simulink model "HVDCMTGW"  (R2025b)
settings: Solver=VariableStepAuto  StartTime=0.0  StopTime=Tsim  FixedStep=5e-5  RelTol=1e-3
PreLoadFcn:
  | SimulationTime = 3.5;
  | HVDCParameters;
  | Tsim = 3.5;
undefined symbols (not defined in the file): base, Base, Connection1, Connection2, Connection3, DiscIntNeverNeededParam, ee_sli_rtmsupport, frt, gcbh, grid, HVDC, lvrt, onshoreGfm, pll, pmsm, PVController, time, Ts, windController, windTransformer, windTurbine
libraries: fl_lib x51, ee_lib x46, nesl_utility x41, simulink x18, eeGeneralControl x12, eeTransforms x6
(part 2 of 4)

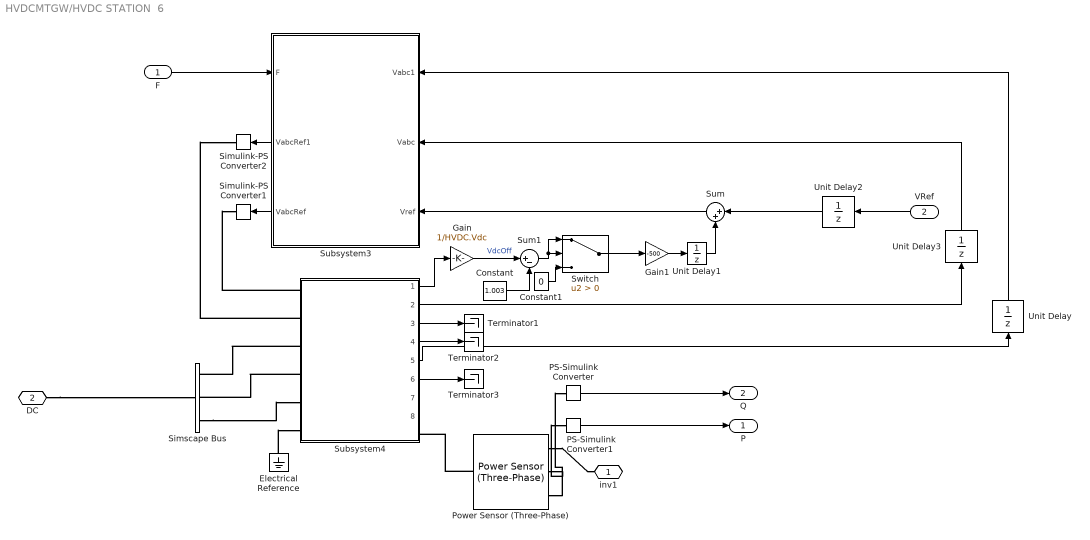
== system HVDCMTGW/HVDC STATION  6 ==
  F : Inport
  VRef : Inport  Port=2
  Constant : Constant  Value=1.003
  Constant1 : Constant  Value=0
  Electrical Reference : fl_lib/Electrical/Electrical Elements/Electrical Reference
  Gain : Gain  Gain=1/HVDC.Vdc
  Gain1 : Gain  Gain=-500
  PS-Simulink Converter : nesl_utility/PS-Simulink Converter  PhysicalDomain=network_engine_domain  SubClassName=ps_output  LeftPortType=input  RightPortType=output  PseudoPeriodic=off  Frequencies=[]  VectorFormat=inherit  Unit=inherit  AffineConversion=off
  PS-Simulink Converter1 : nesl_utility/PS-Simulink Converter  PhysicalDomain=network_engine_domain  SubClassName=ps_output  LeftPortType=input  RightPortType=output  PseudoPeriodic=off  Frequencies=[]  VectorFormat=inherit  Unit=inherit  AffineConversion=off
  Power Sensor (Three-Phase) : ee_lib/Sensors & Transducers/Power Sensor (Three-Phase)  load_type=ee.enum.passive.type_balanced.balanced  f0=60 Hz
      settings: InternalSimscapePortConfiguration="{\"Bottom\":[],\"Left\":[{\"id\":\"N1\",\"label\":\"~1\",\"type\":\"foundation.electrical.three_phase\"}],\"Right\":[{\"id\":\"N2\",\"label\":\"~2\",\"type\":\"foundation.electrical.three_phase\"}],\"Top\":[{\"id\":\"Pm\",\"label\":\"P\",\"type\":\"output\"},{\"id\":\"Qm\",\"label\":\"Q\",\"type\":\"output\"}]}"
  Simscape Bus : SimscapeBus  HierarchyStrings=Connection1;Connection2;Connection3
  Simulink-PS Converter1 : nesl_utility/Simulink-PS Converter  PhysicalDomain=network_engine_domain  SubClassName=ps_input  LeftPortType=input  RightPortType=output  PseudoPeriodic=off  Frequencies=[]  NoiseDistribution=none  NoiseParameters=[]  Unit=1  AffineConversion=off  FilteringAndDerivatives=provide  SimscapeFilterOrder=1  InputFilterTimeConstant=0.001  UdotUserProvided=0
  Simulink-PS Converter2 : nesl_utility/Simulink-PS Converter  PhysicalDomain=network_engine_domain  SubClassName=ps_input  LeftPortType=input  RightPortType=output  PseudoPeriodic=off  Frequencies=[]  NoiseDistribution=none  NoiseParameters=[]  Unit=1  AffineConversion=off  FilteringAndDerivatives=provide  SimscapeFilterOrder=1  InputFilterTimeConstant=0.001  UdotUserProvided=0
  Subsystem3 : Subsystem
      settings: PortSchema="{\"entries\":[{\"content\":{\"sides\":[{\"content\":{\"connectorIds\":[\"In1\",\"In2\",\"In3\"]},\"type\":\"ConnectorPlacement.EquallySpacedRectSide\",\"uuid\":\"fdf47ade-06a3-4164-a0ae-b5ab8f0b8a55\"},{\"content\":{\"connectorIds\":[\"In4\",\"Out1\",\"Out2\"],\"side\":\"RIGHT\"},\"type\":\"ConnectorPlacement.EquallySpacedRectSide\",\"uuid\":\"e0a966ff-b656-4cbf-a7ff-a400da725053\"},{\"content\":{\"side\":\"TOP\"},\"type\":\"ConnectorPlacement.EquallySpacedRectSide\",\"uuid\":\"151062ed-8c36-492f-8148-99554d7644ec\"},{\"content\":{\"side\":\"BOTTOM\"},\"type\":\"ConnectorPlacement.EquallySpacedRectSide\",\"uuid\":\"8f8a2450-c04a-404e-aef9-a0f993b87536\"}]},\"type\":\"ConnectorPlacement.EquallySpacedConnector\",\"uuid\":\"01811104-26cd-432b-92b8-9bb1e91d8204\"}],\"packageUris\":[\"http://schema.mathworks.com/mf0/Connector/R2020b\"],\"version\":\"1.0\"}"
  Subsystem4 : Subsystem  ReferencedSubsystem=HVDCSTATION  c=HVDC.C*0.1  vc=HVDC.Vdc  L=HVDC.L/5  VRated=base.kV1  SRated=Base.MVA_base_new  t=grid.sensorTime  Ts=Ts
  Sum : Sum  Inputs=|++
  Sum1 : Sum  Inputs=|+-
  Switch : Switch  Criteria=u2 > Threshold  SaturateOnIntegerOverflow=off  InputSameDT=off
  Terminator1 : Terminator
  Terminator2 : Terminator
  Terminator3 : Terminator
  Unit Delay{,1..3} (4 alike) : UnitDelay  SampleTime=-1  HasFrameUpgradeWarning=on
  inv1 : PMIOPort  Side=Right
  DC : PMIOPort  Port=2  Side=Left
  P : Outport
  Q : Outport  Port=2
  wires:
  VRef/1 -> Unit Delay2/1
  Subsystem4/4 -> Terminator2/1
  F/1 -> Subsystem3/4(F)
  Subsystem4/2 -> Unit Delay3/1
  Unit Delay/1 -> Subsystem3/1(Vabc1)
  Subsystem4/3 -> Terminator1/1
  Subsystem4/5 -> Unit Delay/1
  Unit Delay3/1 -> Subsystem3/2(Vabc)
  Subsystem4/6 -> Terminator3/1
  Sum/1 -> Subsystem3/3(Vref)
  Subsystem4/1 -> Gain/1
  Unit Delay1/1 -> Sum/2
  Gain1/1 -> Unit Delay1/1
  Gain/1 -> Sum1/1  "VdcOff"
  Constant/1 -> Sum1/2
  Sum1/1 -> Switch/1, Switch/2
  Constant1/1 -> Switch/3
  Switch/1 -> Gain1/1
  PS-Simulink Converter/1 -> Q/1
  PS-Simulink Converter1/1 -> P/1
  Unit Delay2/1 -> Sum/1
  Subsystem3/1(VabcRef1) -> Simulink-PS Converter2/1
  Subsystem3/2(VabcRef) -> Simulink-PS Converter1/1
  connections:
  DC/RConn1 -- Simscape Bus/RConn1
  Subsystem4/LConn3 -- Simscape Bus/LConn1
  Power Sensor (Three-Phase)/LConn1 -- inv1/RConn1
  Power Sensor (Three-Phase)/RConn1 -- Subsystem4/RConn1
  Subsystem4/LConn4 -- Simscape Bus/LConn2
  Simscape Bus/LConn3 -- Subsystem4/LConn5
  Power Sensor (Three-Phase)/LConn3 -- PS-Simulink Converter/LConn1
  Power Sensor (Three-Phase)/LConn2 -- PS-Simulink Converter1/LConn1
  Electrical Reference/LConn1 -- Subsystem4/LConn6
  Subsystem4/LConn1 -- Simulink-PS Converter1/RConn1
  Subsystem4/LConn2 -- Simulink-PS Converter2/RConn1

== system HVDCMTGW/HVDC STATION 1 ==
  QRef1 : Inport
  QRef : Inport  Port=2
  vdcRef : Inport  Port=3
  vdcRef1 : Inport  Port=4
  PS Terminator : fl_lib/Physical Signals/Sinks/PS Terminator
  Simscape Bus : SimscapeBus  HierarchyStrings=Connection1;Connection2;Connection3
  Simulink-PS Converter1 : nesl_utility/Simulink-PS Converter  PhysicalDomain=network_engine_domain  SubClassName=ps_input  LeftPortType=input  RightPortType=output  PseudoPeriodic=off  Frequencies=[]  NoiseDistribution=none  NoiseParameters=[]  Unit=1  AffineConversion=off  FilteringAndDerivatives=provide  SimscapeFilterOrder=1  InputFilterTimeConstant=0.001  UdotUserProvided=0
  Simulink-PS Converter2 : nesl_utility/Simulink-PS Converter  PhysicalDomain=network_engine_domain  SubClassName=ps_input  LeftPortType=input  RightPortType=output  PseudoPeriodic=off  Frequencies=[]  NoiseDistribution=none  NoiseParameters=[]  Unit=1  AffineConversion=off  FilteringAndDerivatives=provide  SimscapeFilterOrder=1  InputFilterTimeConstant=0.001  UdotUserProvided=0
  Subsystem : Subsystem  ReferencedSubsystem=DCVoltageControl  Kppll=PLL.Kp_pll  Kipll=PLL.Ki_pll  frequency=Grid.frequency  initialPhase=0  sampleTime=-1  Kpicd=PVController.Kp_ic*1.02  Kiicd=PVController.Ki_ic*2  Kdicd=.5  Kpicq=PVController.Kp_ic  Kiicq=PVController.Ki_ic*2  Kdicq=.5  Kpv=20  Kiv=1000  Kdv=0  L=HVDC.L*5  iMax=HVDC.Imaxpu  zBase=Base.z_base  mVAbase=Base.MVA_base_new  VdcBase=HVDC.Vdcbase
  Subsystem1 : Subsystem  ReferencedSubsystem=DCVoltageControl  Kppll=PLL.Kp_pll  Kipll=PLL.Ki_pll  frequency=Grid.frequency  initialPhase=0  sampleTime=-1  Kpicd=PVController.Kp_ic*1.02  Kiicd=PVController.Ki_ic*2  Kdicd=0.5  Kpicq=PVController.Kp_ic  Kiicq=PVController.Ki_ic*2  Kdicq=0.5  Kpv=20  Kiv=1000  Kdv=0  L=HVDC.L*5  iMax=HVDC.Imaxpu  zBase=Base.z_base  mVAbase=Base.MVA_base_new  VdcBase=HVDC.Vdcbase
  Subsystem2 : Subsystem  ReferencedSubsystem=HVDCSTATION  c=HVDC.C*0.175  vc=HVDC.Vdc  L=HVDC.L*100  VRated=Base.KV_base_new  SRated=Base.MVA_base_new  t=Grid.sensor_time  Ts=Ts
  Subsystem3 : Subsystem
  Unit Delay1 : UnitDelay  SampleTime=Ts  HasFrameUpgradeWarning=on
  Unit Delay2 : UnitDelay  SampleTime=Ts  HasFrameUpgradeWarning=on
  DC : PMIOPort  Side=Left
  inv1 : PMIOPort  Port=2  Side=Right
  Idc : PMIOPort  Port=3  Side=Left
  wires:
  Unit Delay1/1 -> Simulink-PS Converter1/1
  Unit Delay2/1 -> Simulink-PS Converter2/1
  Subsystem/1 -> Unit Delay2/1
  Subsystem1/1 -> Unit Delay1/1
  vdcRef/1 -> Subsystem/4
  QRef/1 -> Subsystem/5
  vdcRef1/1 -> Subsystem1/4
  QRef1/1 -> Subsystem1/5
  Subsystem2/1 -> Subsystem/1
  Subsystem2/2 -> Subsystem/2
  Subsystem2/3 -> Subsystem/3
  Subsystem2/4 -> Subsystem1/1
  Subsystem2/5 -> Subsystem1/2
  Subsystem2/6 -> Subsystem1/3
  connections:
  Subsystem2/RConn1 -- inv1/RConn1
  Subsystem2/LConn2 -- Simulink-PS Converter1/RConn1
  Subsystem2/LConn1 -- Simulink-PS Converter2/RConn1
  DC/RConn1 -- Simscape Bus/RConn1
  Simscape Bus/LConn2 -- Subsystem3/RConn4 -- Subsystem2/LConn4
  Subsystem3/RConn3 -- Simscape Bus/LConn1
  Subsystem3/LConn1 -- Subsystem2/LConn3
  Idc/RConn1 -- Subsystem3/RConn1
  PS Terminator/LConn1 -- Subsystem3/RConn2
  Simscape Bus/LConn3 -- Subsystem2/LConn5

== system HVDCMTGW/HVDC STATION 2 ==
  QRef1 : Inport
  QRef : Inport  Port=2
  vdcRef1 : Inport  Port=3
  vdcRef : Inport  Port=4
  Bus Selector : BusSelector  OutputSignals=Vmag [pu],f
  Gain : Gain
  PS Terminator : fl_lib/Physical Signals/Sinks/PS Terminator
  Simscape Bus : SimscapeBus  HierarchyStrings=Connection1;Connection2;Connection3
  Simulink-PS Converter1 : nesl_utility/Simulink-PS Converter  PhysicalDomain=network_engine_domain  SubClassName=ps_input  LeftPortType=input  RightPortType=output  PseudoPeriodic=off  Frequencies=[]  NoiseDistribution=none  NoiseParameters=[]  Unit=1  AffineConversion=off  FilteringAndDerivatives=provide  SimscapeFilterOrder=1  InputFilterTimeConstant=0.001  UdotUserProvided=0
  Simulink-PS Converter2 : nesl_utility/Simulink-PS Converter  PhysicalDomain=network_engine_domain  SubClassName=ps_input  LeftPortType=input  RightPortType=output  PseudoPeriodic=off  Frequencies=[]  NoiseDistribution=none  NoiseParameters=[]  Unit=1  AffineConversion=off  FilteringAndDerivatives=provide  SimscapeFilterOrder=1  InputFilterTimeConstant=0.001  UdotUserProvided=0
  Subsystem : Subsystem  ReferencedSubsystem=DCVoltageControl  Kppll=PLL.Kp_pll  Kipll=PLL.Ki_pll  frequency=Grid.frequency  initialPhase=0  sampleTime=-1  Kpicd=PVController.Kp_ic*1.02  Kiicd=PVController.Ki_ic*2  Kdicd=.5  Kpicq=PVController.Kp_ic  Kiicq=PVController.Ki_ic*2  Kdicq=.5  Kpv=20  Kiv=1000  Kdv=0  L=HVDC.L*5  iMax=HVDC.Imaxpu  zBase=Base.z_base  mVAbase=Base.MVA_base_new  VdcBase=HVDC.Vdcbase
  Subsystem1 : Subsystem  ReferencedSubsystem=DCVoltageControl  Kppll=PLL.Kp_pll  Kipll=PLL.Ki_pll  frequency=Grid.frequency  initialPhase=0  sampleTime=-1  Kpicd=PVController.Kp_ic*1.02  Kiicd=PVController.Ki_ic*2  Kdicd=0.5  Kpicq=PVController.Kp_ic  Kiicq=PVController.Ki_ic*2  Kdicq=0.5  Kpv=20  Kiv=1000  Kdv=0  L=HVDC.L*5  iMax=HVDC.Imaxpu  zBase=Base.z_base  mVAbase=Base.MVA_base_new  VdcBase=HVDC.Vdcbase
  Subsystem2 : Subsystem  ReferencedSubsystem=HVDCSTATION  c=HVDC.C*0.175  vc=HVDC.Vdc  L=HVDC.L*100  VRated=Base.KV_base_new  SRated=Base.MVA_base_new  t=Grid.sensor_time  Ts=Ts
  Subsystem3 : Subsystem
  Terminator : Terminator
  Terminator1 : Terminator
  To Workspace1 : ToWorkspace  VariableName=f  SaveFormat=Timeseries  SampleTime=-1
  To Workspace3 : ToWorkspace  VariableName=Vmag  SaveFormat=Timeseries  SampleTime=-1
  Unit Delay1 : UnitDelay  SampleTime=Ts  HasFrameUpgradeWarning=on
  Unit Delay2 : UnitDelay  SampleTime=Ts  HasFrameUpgradeWarning=on
  Idc : PMIOPort  Side=Left
  DC : PMIOPort  Port=2  Side=Left
  inv1 : PMIOPort  Port=3  Side=Right
  wires:
  Unit Delay1/1 -> Simulink-PS Converter1/1
  Unit Delay2/1 -> Simulink-PS Converter2/1
  Subsystem/1 -> Unit Delay2/1
  Subsystem1/1 -> Unit Delay1/1
  vdcRef/1 -> Subsystem/4
  QRef/1 -> Subsystem/5
  vdcRef1/1 -> Subsystem1/4
  QRef1/1 -> Subsystem1/5
  Subsystem2/1 -> Subsystem/1
  Subsystem2/2 -> Subsystem/2
  Subsystem2/3 -> Subsystem/3
  Subsystem2/4 -> Subsystem1/1
  Subsystem2/5 -> Subsystem1/2
  Subsystem2/6 -> Subsystem1/3
  Subsystem/2 -> Bus Selector/1
  Bus Selector/1 -> To Workspace3/1, Terminator/1  "<Vmag [pu]>"
  Bus Selector/2 -> Gain/1, Terminator1/1  "<f>"
  Gain/1 -> To Workspace1/1
  connections:
  Subsystem2/RConn1 -- inv1/RConn1
  Subsystem2/LConn2 -- Simulink-PS Converter1/RConn1
  Subsystem2/LConn1 -- Simulink-PS Converter2/RConn1
  Simscape Bus/LConn3 -- Subsystem2/LConn5
  DC/RConn1 -- Simscape Bus/RConn1
  Simscape Bus/LConn2 -- Subsystem3/RConn4 -- Subsystem2/LConn4
  Subsystem3/RConn3 -- Simscape Bus/LConn1
  Idc/RConn1 -- Subsystem3/RConn1
  Subsystem3/LConn1 -- Subsystem2/LConn3
  PS Terminator/LConn1 -- Subsystem3/RConn2

== system HVDCMTGW/HVDC STATION 3 ==
  QRef : Inport
  QRef1 : Inport  Port=2
  vdcRef : Inport  Port=3
  vdcRef1 : Inport  Port=4
  GFL Control : Subsystem  VariantControl=Choice==1
      mask Display:
      | text(40,10, 'Grid Following');
      | image('HVDCstation1.png', [0,2,12,2,80,80]);
  GFM Control : Subsystem  VariantControl=Choice==2
      mask Display:
      | text(40,10, 'Grid Forming');
      | image('HVDCstation1.png', [0,2,12,2,80,80]);
  Idc : PMIOPort  Side=Left
  DC : PMIOPort  Port=2  Side=Left
  inv1 : PMIOPort  Port=3  Side=Right

== system HVDCMTGW/Subsystem ==
  Pm : Inport
  Pref : Inport  Port=2
  Constant : Constant  Value=f
  Gain : Gain  Gain=kp
  Lead-Lag (Discrete or Continuous) : eeGeneralControl/Lead-Lag (Discrete or Continuous)  T1=0  T2=t  B=inf  A=-inf  init_option=Inherited from block input  x0=0  Ts=-1
      settings: LibrarySourceBlock=|
      | ee_sl_lib/General Control/Lead-Lag
      | (Discrete or Continuous)
  Sum : Sum  Inputs=|+-
  Sum1 : Sum  Inputs=|++
  f : Outport
  wires:
  Pref/1 -> Sum/1
  Sum/1 -> Gain/1
  Pm/1 -> Lead-Lag (Discrete or Continuous)/1
  Constant/1 -> Sum1/2
  Sum1/1 -> f/1
  Lead-Lag (Discrete or Continuous)/1 -> Sum/2
  Gain/1 -> Sum1/1

== system HVDCMTGW/Subsystem1 ==
  Qm : Inport
  Qref : Inport  Port=2
  Constant : Constant  Value=V
  Gain : Gain  Gain=kq
  Lead-Lag (Discrete or Continuous) : eeGeneralControl/Lead-Lag (Discrete or Continuous)  T1=0  T2=t  B=inf  A=-inf  init_option=Inherited from block input  x0=0  Ts=-1
      settings: LibrarySourceBlock=|
      | ee_sl_lib/General Control/Lead-Lag
      | (Discrete or Continuous)
  Sum : Sum  Inputs=|+-
  Sum1 : Sum  Inputs=|++
  V : Outport
  wires:
  Qref/1 -> Sum/1
  Sum/1 -> Gain/1
  Qm/1 -> Lead-Lag (Discrete or Continuous)/1
  Constant/1 -> Sum1/2
  Sum1/1 -> V/1
  Lead-Lag (Discrete or Continuous)/1 -> Sum/2
  Gain/1 -> Sum1/1

== system HVDCMTGW/Subsystem2 ==
  Pm : Inport
  Pref : Inport  Port=2
  Constant : Constant  Value=f
  Gain : Gain  Gain=kp
  Lead-Lag (Discrete or Continuous) : eeGeneralControl/Lead-Lag (Discrete or Continuous)  T1=0  T2=t  B=inf  A=-inf  init_option=Inherited from block input  x0=0  Ts=-1
      settings: LibrarySourceBlock=|
      | ee_sl_lib/General Control/Lead-Lag
      | (Discrete or Continuous)
  Sum : Sum  Inputs=|+-
  Sum1 : Sum  Inputs=|++
  f : Outport
  wires:
  Pref/1 -> Sum/1
  Sum/1 -> Gain/1
  Pm/1 -> Lead-Lag (Discrete or Continuous)/1
  Constant/1 -> Sum1/2
  Sum1/1 -> f/1
  Gain/1 -> Sum1/1
  Lead-Lag (Discrete or Continuous)/1 -> Sum/2

== system HVDCMTGW/Subsystem3 ==
  Qm : Inport
  Qref : Inport  Port=2
  Constant : Constant  Value=V
  Gain : Gain  Gain=kq
  Lead-Lag (Discrete or Continuous) : eeGeneralControl/Lead-Lag (Discrete or Continuous)  T1=0  T2=t  B=inf  A=-inf  init_option=Inherited from block input  x0=0  Ts=-1
      settings: LibrarySourceBlock=|
      | ee_sl_lib/General Control/Lead-Lag
      | (Discrete or Continuous)
  Sum : Sum  Inputs=|+-
  Sum1 : Sum  Inputs=|++
  V : Outport
  wires:
  Qref/1 -> Sum/1
  Sum/1 -> Gain/1
  Constant/1 -> Sum1/2
  Qm/1 -> Lead-Lag (Discrete or Continuous)/1
  Gain/1 -> Sum1/1
  Sum1/1 -> V/1
  Lead-Lag (Discrete or Continuous)/1 -> Sum/2

== system HVDCMTGW/Wind Farm 1 ==
  AC Cable (Three-Phase) : ee_lib/Passive/Lines/AC Cable (Three-Phase)  l=2 km  gmr=5 mm  srad=10 mm  cablerad=20 mm  Dab=25 mm  formation=1  Ra=1 Ohm/km  Rs=10 Ohm/km  epsr=2.4  epsr_env=1  prm=1  f=60 Hz  rho=100 Ohm*m  De=1 km  Rg=0.1 Ohm/km
      settings: InternalSimscapePortConfiguration="{\"Bottom\":[],\"Left\":[{\"id\":\"S1\",\"label\":\"~S1\",\"type\":\"foundation.electrical.three_phase\"},{\"id\":\"N1\",\"label\":\"~N1\",\"type\":\"foundation.electrical.three_phase\"},{\"id\":\"g1\",\"label\":\"g1\",\"type\":\"foundation.electrical.electrical\"}],\"Right\":[{\"id\":\"S2\",\"label\":\"~S2\",\"type\":\"foundation.electrical.three_phase\"},{\"id\":\"N2\",\"label\":\"~N2\",\"type\":\"foundation.electrical.three_phase\"},{\"id\":\"g2\",\"label\":\"g2\",\"type\":\"foundation.electrical.electrical\"}],\"Top\":[]}"
  Electrical Reference : fl_lib/Electrical/Electrical Elements/Electrical Reference
  Electrical Reference1 : fl_lib/Electrical/Electrical Elements/Electrical Reference
  PLL & Measurements : Subsystem
      settings: PortSchema="{\"entries\":[{\"content\":{\"sides\":[{\"content\":{\"connectorIds\":[\"Out1\",\"In1\",\"In2\"]},\"type\":\"ConnectorPlacement.EquallySpacedRectSide\",\"uuid\":\"76485780-20fe-4fcf-8224-69648da6ed2a\"},{\"content\":{\"side\":\"RIGHT\"},\"type\":\"ConnectorPlacement.EquallySpacedRectSide\",\"uuid\":\"f19a6390-e634-42c7-8d46-4cd80cbab182\"},{\"content\":{\"side\":\"TOP\"},\"type\":\"ConnectorPlacement.EquallySpacedRectSide\",\"uuid\":\"87682f72-1844-428e-be70-ad7ca3191ee3\"}]},\"type\":\"ConnectorPlacement.EquallySpacedConnector\",\"uuid\":\"f2136b07-48ec-402b-adb3-18c0bac2157c\"}],\"packageUris\":[\"http://schema.mathworks.com/mf0/Connector/R2020b\"],\"version\":\"1.0\"}"
      mask Display: image('measurements.png'); % Use "Edit Image" on toolstrip to change.
  Wind Farm : Subsystem  Variant=on  mask{Choice1=Abstract}
      mask prompts: Choice1 "Wind Farm Model"
  abc : PMIOPort  Side=Right
  wires:
  PLL & Measurements/1(Vbus) -> Wind Farm/1(Vbus)
  Wind Farm/1(Vabc) -> PLL & Measurements/1(V)
  Wind Farm/2(Iabc) -> PLL & Measurements/2(Ig)
  connections:
  Electrical Reference/LConn1 -- AC Cable (Three-Phase)/LConn3
  Electrical Reference1/LConn1 -- AC Cable (Three-Phase)/RConn3
  AC Cable (Three-Phase)/LConn2 -- abc/RConn1
  Wind Farm/RConn1 -- Wind Farm/RConn2 -- AC Cable (Three-Phase)/RConn2

== system HVDCMTGW/Wind Farm 2 ==
  AC Cable (Three-Phase) : ee_lib/Passive/Lines/AC Cable (Three-Phase)  l=2 km  gmr=5 mm  srad=10 mm  cablerad=20 mm  Dab=25 mm  formation=1  Ra=1 Ohm/km  Rs=10 Ohm/km  epsr=2.4  epsr_env=1  prm=1  f=60 Hz  rho=100 Ohm*m  De=1 km  Rg=0.1 Ohm/km
      settings: InternalSimscapePortConfiguration="{\"Bottom\":[],\"Left\":[{\"id\":\"S1\",\"label\":\"~S1\",\"type\":\"foundation.electrical.three_phase\"},{\"id\":\"N1\",\"label\":\"~N1\",\"type\":\"foundation.electrical.three_phase\"},{\"id\":\"g1\",\"label\":\"g1\",\"type\":\"foundation.electrical.electrical\"}],\"Right\":[{\"id\":\"S2\",\"label\":\"~S2\",\"type\":\"foundation.electrical.three_phase\"},{\"id\":\"N2\",\"label\":\"~N2\",\"type\":\"foundation.electrical.three_phase\"},{\"id\":\"g2\",\"label\":\"g2\",\"type\":\"foundation.electrical.electrical\"}],\"Top\":[]}"
  AC Cable (Three-Phase)1 : ee_lib/Passive/Lines/AC Cable (Three-Phase)  l=5 km  gmr=5 mm  srad=10 mm  cablerad=20 mm  Dab=25 mm  formation=1  Ra=1 Ohm/km  Rs=10 Ohm/km  epsr=2.4  epsr_env=1  prm=1  f=60 Hz  rho=100 Ohm*m  De=1 km  Rg=0.1 Ohm/km
      settings: InternalSimscapePortConfiguration="{\"Bottom\":[],\"Left\":[{\"id\":\"S1\",\"label\":\"~S1\",\"type\":\"foundation.electrical.three_phase\"},{\"id\":\"N1\",\"label\":\"~N1\",\"type\":\"foundation.electrical.three_phase\"},{\"id\":\"g1\",\"label\":\"g1\",\"type\":\"foundation.electrical.electrical\"}],\"Right\":[{\"id\":\"S2\",\"label\":\"~S2\",\"type\":\"foundation.electrical.three_phase\"},{\"id\":\"N2\",\"label\":\"~N2\",\"type\":\"foundation.electrical.three_phase\"},{\"id\":\"g2\",\"label\":\"g2\",\"type\":\"foundation.electrical.electrical\"}],\"Top\":[]}"
  Electrical Reference{,1..3} (4 alike) : fl_lib/Electrical/Electrical Elements/Electrical Reference
  PLL & Measurements : Subsystem
      settings: PortSchema="{\"entries\":[{\"content\":{\"sides\":[{\"content\":{\"connectorIds\":[\"Out1\",\"In1\",\"In2\"]},\"type\":\"ConnectorPlacement.EquallySpacedRectSide\",\"uuid\":\"76485780-20fe-4fcf-8224-69648da6ed2a\"},{\"content\":{\"side\":\"RIGHT\"},\"type\":\"ConnectorPlacement.EquallySpacedRectSide\",\"uuid\":\"f19a6390-e634-42c7-8d46-4cd80cbab182\"},{\"content\":{\"side\":\"TOP\"},\"type\":\"ConnectorPlacement.EquallySpacedRectSide\",\"uuid\":\"87682f72-1844-428e-be70-ad7ca3191ee3\"}]},\"type\":\"ConnectorPlacement.EquallySpacedConnector\",\"uuid\":\"f2136b07-48ec-402b-adb3-18c0bac2157c\"}],\"packageUris\":[\"http://schema.mathworks.com/mf0/Connector/R2020b\"],\"version\":\"1.0\"}"
      mask Display: image('measurements.png'); % Use "Edit Image" on toolstrip to change.
  Wind Farm : Subsystem  Variant=on  mask{Choice1=Abstract}
      mask prompts: Choice1 "Wind Farm Model"
  abc1 : PMIOPort  Side=Right
  abc : PMIOPort  Port=2  Side=Right
  wires:
  PLL & Measurements/1(Vbus) -> Wind Farm/1(Vbus)
  Wind Farm/1(Vabc) -> PLL & Measurements/1(V)
  Wind Farm/2(Iabc) -> PLL & Measurements/2(Ig)
  connections:
  Electrical Reference/LConn1 -- AC Cable (Three-Phase)/LConn3
  Electrical Reference1/LConn1 -- AC Cable (Three-Phase)/RConn3
  AC Cable (Three-Phase)/LConn2 -- abc/RConn1
  Electrical Reference2/LConn1 -- AC Cable (Three-Phase)1/LConn3
  Electrical Reference3/LConn1 -- AC Cable (Three-Phase)1/RConn3
  abc1/RConn1 -- AC Cable (Three-Phase)1/LConn2
  Wind Farm/RConn1 -- AC Cable (Three-Phase)/RConn2
  AC Cable (Three-Phase)1/RConn2 -- Wind Farm/RConn2

== system HVDCMTGW/HVDC Network/DC Line 10 km ==
  Inductor : ee_lib/Passive/Inductor  l=Ldc*l H  enable_L_tol=ee.enum.toleranceApplication.none  L_tol=20  tol_distribution=ee.enum.toleranceDistribution.uniform  nSigma=4  r=0 Ohm  g=1e-9 1/Ohm  enable_operating_limits=ee.enum.enable.no  operating_limit_action=ee.enum.passive.reportOpLim.warn  max_working_current=1 A  power_rating=1 W  i_L_specify=off  i_L_priority=High  i_L=0 A  i_L_nominal_specify=off  i_L_nominal_value=1  i_L_nominal_unit=A
  Inductor2 : ee_lib/Passive/Inductor  l=Ldc*l H  enable_L_tol=ee.enum.toleranceApplication.none  L_tol=20  tol_distribution=ee.enum.toleranceDistribution.uniform  nSigma=4  r=0 Ohm  g=1e-9 1/Ohm  enable_operating_limits=ee.enum.enable.no  operating_limit_action=ee.enum.passive.reportOpLim.warn  max_working_current=1 A  power_rating=1 W  i_L_specify=off  i_L_priority=High  i_L=0 A  i_L_nominal_specify=off  i_L_nominal_value=1  i_L_nominal_unit=A
  Resistor : fl_lib/Electrical/Electrical Elements/Resistor  R=rdc*l Ohm  i_specify=off  i_priority=None  i=0 A  i_nominal_specify=off  i_nominal_value=1  i_nominal_unit=A  v_specify=off  v_priority=None  v=0 V  v_nominal_specify=off  v_nominal_value=1  v_nominal_unit=V
  Resistor1 : fl_lib/Electrical/Electrical Elements/Resistor  R=rdc*l Ohm  i_specify=off  i_priority=None  i=0 A  i_nominal_specify=off  i_nominal_value=1  i_nominal_unit=A  v_specify=off  v_priority=None  v=0 V  v_nominal_specify=off  v_nominal_value=1  v_nominal_unit=V
  Resistor2 : fl_lib/Electrical/Electrical Elements/Resistor  R=rn*l Ohm  i_specify=off  i_priority=None  i=0 A  i_nominal_specify=off  i_nominal_value=1  i_nominal_unit=A  v_specify=off  v_priority=None  v=0 V  v_nominal_specify=off  v_nominal_value=1  v_nominal_unit=V
  Conn1 : PMIOPort  Side=Right
  Conn2 : PMIOPort  Port=2  Side=Left
  Conn3 : PMIOPort  Port=3  Side=Right
  Conn4 : PMIOPort  Port=4  Side=Left
  Conn5 : PMIOPort  Port=5  Side=Right
  Conn6 : PMIOPort  Port=6  Side=Left
  connections:
  Resistor1/LConn1 -- Conn6/RConn1
  Inductor/LConn1 -- Resistor/RConn1
  Inductor2/LConn1 -- Resistor1/RConn1
  Resistor2/RConn1 -- Conn3/RConn1
  Resistor2/LConn1 -- Conn4/RConn1
  Resistor/LConn1 -- Conn2/RConn1
  Inductor/RConn1 -- Conn1/RConn1
  Inductor2/RConn1 -- Conn5/RConn1

== system HVDCMTGW/HVDC Network/DC Line 125 km ==
  Inductor : ee_lib/Passive/Inductor  l=Ldc*l H  enable_L_tol=ee.enum.toleranceApplication.none  L_tol=20  tol_distribution=ee.enum.toleranceDistribution.uniform  nSigma=4  r=0 Ohm  g=1e-9 1/Ohm  enable_operating_limits=ee.enum.enable.no  operating_limit_action=ee.enum.passive.reportOpLim.warn  max_working_current=1 A  power_rating=1 W  i_L_specify=off  i_L_priority=High  i_L=0 A  i_L_nominal_specify=off  i_L_nominal_value=1  i_L_nominal_unit=A
  Inductor2 : ee_lib/Passive/Inductor  l=Ldc*l H  enable_L_tol=ee.enum.toleranceApplication.none  L_tol=20  tol_distribution=ee.enum.toleranceDistribution.uniform  nSigma=4  r=0 Ohm  g=1e-9 1/Ohm  enable_operating_limits=ee.enum.enable.no  operating_limit_action=ee.enum.passive.reportOpLim.warn  max_working_current=1 A  power_rating=1 W  i_L_specify=off  i_L_priority=High  i_L=0 A  i_L_nominal_specify=off  i_L_nominal_value=1  i_L_nominal_unit=A
  Resistor : fl_lib/Electrical/Electrical Elements/Resistor  R=rdc*l Ohm  i_specify=off  i_priority=None  i=0 A  i_nominal_specify=off  i_nominal_value=1  i_nominal_unit=A  v_specify=off  v_priority=None  v=0 V  v_nominal_specify=off  v_nominal_value=1  v_nominal_unit=V
  Resistor1 : fl_lib/Electrical/Electrical Elements/Resistor  R=rdc*l Ohm  i_specify=off  i_priority=None  i=0 A  i_nominal_specify=off  i_nominal_value=1  i_nominal_unit=A  v_specify=off  v_priority=None  v=0 V  v_nominal_specify=off  v_nominal_value=1  v_nominal_unit=V
  Resistor2 : fl_lib/Electrical/Electrical Elements/Resistor  R=rn*l Ohm  i_specify=off  i_priority=None  i=0 A  i_nominal_specify=off  i_nominal_value=1  i_nominal_unit=A  v_specify=off  v_priority=None  v=0 V  v_nominal_specify=off  v_nominal_value=1  v_nominal_unit=V
  Conn1 : PMIOPort  Side=Right
  Conn2 : PMIOPort  Port=2  Side=Left
  Conn3 : PMIOPort  Port=3  Side=Right
  Conn4 : PMIOPort  Port=4  Side=Left
  Conn5 : PMIOPort  Port=5  Side=Right
  Conn6 : PMIOPort  Port=6  Side=Left
  connections:
  Resistor1/LConn1 -- Conn6/RConn1
  Inductor/LConn1 -- Resistor/RConn1
  Inductor2/LConn1 -- Resistor1/RConn1
  Resistor2/RConn1 -- Conn3/RConn1
  Resistor2/LConn1 -- Conn4/RConn1
  Resistor/LConn1 -- Conn2/RConn1
  Inductor/RConn1 -- Conn1/RConn1
  Inductor2/RConn1 -- Conn5/RConn1

== system HVDCMTGW/HVDC Network/DC Line 200 km ==
  Inductor : ee_lib/Passive/Inductor  l=Ldc*l H  enable_L_tol=ee.enum.toleranceApplication.none  L_tol=20  tol_distribution=ee.enum.toleranceDistribution.uniform  nSigma=4  r=0 Ohm  g=1e-9 1/Ohm  enable_operating_limits=ee.enum.enable.no  operating_limit_action=ee.enum.passive.reportOpLim.warn  max_working_current=1 A  power_rating=1 W  i_L_specify=off  i_L_priority=High  i_L=0 A  i_L_nominal_specify=off  i_L_nominal_value=1  i_L_nominal_unit=A
  Inductor2 : ee_lib/Passive/Inductor  l=Ldc*l H  enable_L_tol=ee.enum.toleranceApplication.none  L_tol=20  tol_distribution=ee.enum.toleranceDistribution.uniform  nSigma=4  r=0 Ohm  g=1e-9 1/Ohm  enable_operating_limits=ee.enum.enable.no  operating_limit_action=ee.enum.passive.reportOpLim.warn  max_working_current=1 A  power_rating=1 W  i_L_specify=off  i_L_priority=High  i_L=0 A  i_L_nominal_specify=off  i_L_nominal_value=1  i_L_nominal_unit=A
  Resistor : fl_lib/Electrical/Electrical Elements/Resistor  R=rdc*l Ohm  i_specify=off  i_priority=None  i=0 A  i_nominal_specify=off  i_nominal_value=1  i_nominal_unit=A  v_specify=off  v_priority=None  v=0 V  v_nominal_specify=off  v_nominal_value=1  v_nominal_unit=V
  Resistor1 : fl_lib/Electrical/Electrical Elements/Resistor  R=rdc*l Ohm  i_specify=off  i_priority=None  i=0 A  i_nominal_specify=off  i_nominal_value=1  i_nominal_unit=A  v_specify=off  v_priority=None  v=0 V  v_nominal_specify=off  v_nominal_value=1  v_nominal_unit=V
  Resistor2 : fl_lib/Electrical/Electrical Elements/Resistor  R=rn*l Ohm  i_specify=off  i_priority=None  i=0 A  i_nominal_specify=off  i_nominal_value=1  i_nominal_unit=A  v_specify=off  v_priority=None  v=0 V  v_nominal_specify=off  v_nominal_value=1  v_nominal_unit=V
  Conn1 : PMIOPort  Side=Right
  Conn2 : PMIOPort  Port=2  Side=Left
  Conn3 : PMIOPort  Port=3  Side=Right
  Conn4 : PMIOPort  Port=4  Side=Left
  Conn5 : PMIOPort  Port=5  Side=Right
  Conn6 : PMIOPort  Port=6  Side=Left
  connections:
  Resistor1/LConn1 -- Conn6/RConn1
  Inductor/LConn1 -- Resistor/RConn1
  Inductor2/LConn1 -- Resistor1/RConn1
  Resistor2/RConn1 -- Conn3/RConn1
  Resistor2/LConn1 -- Conn4/RConn1
  Resistor/LConn1 -- Conn2/RConn1
  Inductor/RConn1 -- Conn1/RConn1
  Inductor2/RConn1 -- Conn5/RConn1

== system HVDCMTGW/HVDC Network/DC Line 205 km ==
  Inductor : ee_lib/Passive/Inductor  l=Ldc*l H  enable_L_tol=ee.enum.toleranceApplication.none  L_tol=20  tol_distribution=ee.enum.toleranceDistribution.uniform  nSigma=4  r=0 Ohm  g=1e-9 1/Ohm  enable_operating_limits=ee.enum.enable.no  operating_limit_action=ee.enum.passive.reportOpLim.warn  max_working_current=1 A  power_rating=1 W  i_L_specify=off  i_L_priority=High  i_L=0 A  i_L_nominal_specify=off  i_L_nominal_value=1  i_L_nominal_unit=A
  Inductor2 : ee_lib/Passive/Inductor  l=Ldc*l H  enable_L_tol=ee.enum.toleranceApplication.none  L_tol=20  tol_distribution=ee.enum.toleranceDistribution.uniform  nSigma=4  r=0 Ohm  g=1e-9 1/Ohm  enable_operating_limits=ee.enum.enable.no  operating_limit_action=ee.enum.passive.reportOpLim.warn  max_working_current=1 A  power_rating=1 W  i_L_specify=off  i_L_priority=High  i_L=0 A  i_L_nominal_specify=off  i_L_nominal_value=1  i_L_nominal_unit=A
  Resistor : fl_lib/Electrical/Electrical Elements/Resistor  R=rdc*l Ohm  i_specify=off  i_priority=None  i=0 A  i_nominal_specify=off  i_nominal_value=1  i_nominal_unit=A  v_specify=off  v_priority=None  v=0 V  v_nominal_specify=off  v_nominal_value=1  v_nominal_unit=V
  Resistor1 : fl_lib/Electrical/Electrical Elements/Resistor  R=rdc*l Ohm  i_specify=off  i_priority=None  i=0 A  i_nominal_specify=off  i_nominal_value=1  i_nominal_unit=A  v_specify=off  v_priority=None  v=0 V  v_nominal_specify=off  v_nominal_value=1  v_nominal_unit=V
  Resistor2 : fl_lib/Electrical/Electrical Elements/Resistor  R=rn*l Ohm  i_specify=off  i_priority=None  i=0 A  i_nominal_specify=off  i_nominal_value=1  i_nominal_unit=A  v_specify=off  v_priority=None  v=0 V  v_nominal_specify=off  v_nominal_value=1  v_nominal_unit=V
  Conn1 : PMIOPort  Side=Right
  Conn2 : PMIOPort  Port=2  Side=Left
  Conn3 : PMIOPort  Port=3  Side=Right
  Conn4 : PMIOPort  Port=4  Side=Left
  Conn5 : PMIOPort  Port=5  Side=Right
  Conn6 : PMIOPort  Port=6  Side=Left
  connections:
  Resistor1/LConn1 -- Conn6/RConn1
  Inductor/LConn1 -- Resistor/RConn1
  Inductor2/LConn1 -- Resistor1/RConn1
  Resistor2/RConn1 -- Conn3/RConn1
  Resistor2/LConn1 -- Conn4/RConn1
  Resistor/LConn1 -- Conn2/RConn1
  Inductor/RConn1 -- Conn1/RConn1
  Inductor2/RConn1 -- Conn5/RConn1

== system HVDCMTGW/HVDC STATION  4/Subsystem3 ==
  Vabc1 : Inport
  Vabc : Inport  Port=2
  Vref : Inport  Port=3
  F : Inport  Port=4
  F1 : InportShadow  Port=4
  Subsystem1 : Subsystem  ReferencedSubsystem=WFController  Kpv=offshoregfm.kvp  Kiv=offshoregfm.kvi  Kpicd=offshoregfm.kip  Kiicd=offshoregfm.kii  Kpicq=offshoregfm.kip  Kiicq=offshoregfm.kii  mVAbase=base.mVA  frequency=Grid.frequency  zBase=base.z  iMax=offshoregfm.Imax  L=HVDC.L/5  Kv=base.kV1
      settings: PortSchema="{\"entries\":[{\"content\":{\"sides\":[{\"content\":{\"connectorIds\":[\"In1\"]},\"type\":\"ConnectorPlacement.EquallySpacedRectSide\",\"uuid\":\"46af9a47-930e-4d26-bbce-c3520b6c2749\"},{\"content\":{\"connectorIds\":[\"Out1\"],\"side\":\"RIGHT\"},\"type\":\"ConnectorPlacement.EquallySpacedRectSide\",\"uuid\":\"6339fe7c-3981-41e7-9f19-cda16be41a14\"},{\"content\":{\"side\":\"TOP\"},\"type\":\"ConnectorPlacement.EquallySpacedRectSide\",\"uuid\":\"d1729033-563f-49aa-8053-bb4cbe37e0ab\"},{\"content\":{\"connectorIds\":[\"In2\",\"In3\"],\"side\":\"BOTTOM\"},\"type\":\"ConnectorPlacement.EquallySpacedRectSide\",\"uuid\":\"30ea6182-355c-4132-b992-4839827195ad\"}]},\"type\":\"ConnectorPlacement.EquallySpacedConnector\",\"uuid\":\"fc0bd660-6248-4e50-8baf-5497ce638304\"}],\"packageUris\":[\"http://schema.mathworks.com/mf0/Connector/R2020b\"],\"version\":\"1.0\"}"
  Subsystem2 : Subsystem  ReferencedSubsystem=WFController  Kpv=offshoregfm.kvp  Kiv=offshoregfm.kvi  Kpicd=offshoregfm.kip  Kiicd=offshoregfm.kii  Kpicq=offshoregfm.kip  Kiicq=offshoregfm.kii  mVAbase=base.mVA  frequency=Grid.frequency  zBase=base.z  iMax=offshoregfm.Imax  L=HVDC.L/5  Kv=base.kV1
      settings: PortSchema="{\"entries\":[{\"content\":{\"sides\":[{\"content\":{\"connectorIds\":[\"In1\"]},\"type\":\"ConnectorPlacement.EquallySpacedRectSide\",\"uuid\":\"46af9a47-930e-4d26-bbce-c3520b6c2749\"},{\"content\":{\"connectorIds\":[\"Out1\"],\"side\":\"RIGHT\"},\"type\":\"ConnectorPlacement.EquallySpacedRectSide\",\"uuid\":\"6339fe7c-3981-41e7-9f19-cda16be41a14\"},{\"content\":{\"side\":\"TOP\"},\"type\":\"ConnectorPlacement.EquallySpacedRectSide\",\"uuid\":\"d1729033-563f-49aa-8053-bb4cbe37e0ab\"},{\"content\":{\"connectorIds\":[\"In2\",\"In3\"],\"side\":\"BOTTOM\"},\"type\":\"ConnectorPlacement.EquallySpacedRectSide\",\"uuid\":\"30ea6182-355c-4132-b992-4839827195ad\"}]},\"type\":\"ConnectorPlacement.EquallySpacedConnector\",\"uuid\":\"fc0bd660-6248-4e50-8baf-5497ce638304\"}],\"packageUris\":[\"http://schema.mathworks.com/mf0/Connector/R2020b\"],\"version\":\"1.0\"}"
  Vref1 : InportShadow  Port=3
  VabcRef1 : Outport
  VabcRef : Outport  Port=2
  wires:
  Vabc/1 -> Subsystem1/1
  Vref/1 -> Subsystem1/3
  F/1 -> Subsystem1/2
  Vabc1/1 -> Subsystem2/1
  F1/1 -> Subsystem2/2
  Vref1/1 -> Subsystem2/3
  Subsystem1/1 -> VabcRef/1
  Subsystem2/1 -> VabcRef1/1

== system HVDCMTGW/HVDC STATION  5/Subsystem3 ==
  Vabc1 : Inport
  Vabc : Inport  Port=2
  Vref : Inport  Port=3
  F : Inport  Port=4
  F1 : InportShadow  Port=4
  Subsystem1 : Subsystem  ReferencedSubsystem=WFController  Kpv=offshoregfm.kvp  Kiv=offshoregfm.kvi  Kpicd=offshoregfm.kip  Kiicd=offshoregfm.kii  Kpicq=offshoregfm.kip  Kiicq=offshoregfm.kii  mVAbase=base.mVA  frequency=Grid.frequency  zBase=base.z  iMax=offshoregfm.Imax  L=HVDC.L/5  Kv=base.kV1
      settings: PortSchema="{\"entries\":[{\"content\":{\"sides\":[{\"content\":{\"connectorIds\":[\"In1\"]},\"type\":\"ConnectorPlacement.EquallySpacedRectSide\",\"uuid\":\"46af9a47-930e-4d26-bbce-c3520b6c2749\"},{\"content\":{\"connectorIds\":[\"Out1\"],\"side\":\"RIGHT\"},\"type\":\"ConnectorPlacement.EquallySpacedRectSide\",\"uuid\":\"6339fe7c-3981-41e7-9f19-cda16be41a14\"},{\"content\":{\"side\":\"TOP\"},\"type\":\"ConnectorPlacement.EquallySpacedRectSide\",\"uuid\":\"d1729033-563f-49aa-8053-bb4cbe37e0ab\"},{\"content\":{\"connectorIds\":[\"In2\",\"In3\"],\"side\":\"BOTTOM\"},\"type\":\"ConnectorPlacement.EquallySpacedRectSide\",\"uuid\":\"30ea6182-355c-4132-b992-4839827195ad\"}]},\"type\":\"ConnectorPlacement.EquallySpacedConnector\",\"uuid\":\"fc0bd660-6248-4e50-8baf-5497ce638304\"}],\"packageUris\":[\"http://schema.mathworks.com/mf0/Connector/R2020b\"],\"version\":\"1.0\"}"
  Subsystem2 : Subsystem  ReferencedSubsystem=WFController  Kpv=offshoregfm.kvp  Kiv=offshoregfm.kvi  Kpicd=offshoregfm.kip  Kiicd=offshoregfm.kii  Kpicq=offshoregfm.kip  Kiicq=offshoregfm.kii  mVAbase=base.mVA  frequency=Grid.frequency  zBase=base.z  iMax=offshoregfm.Imax  L=HVDC.L/5  Kv=base.kV1
      settings: PortSchema="{\"entries\":[{\"content\":{\"sides\":[{\"content\":{\"connectorIds\":[\"In1\"]},\"type\":\"ConnectorPlacement.EquallySpacedRectSide\",\"uuid\":\"46af9a47-930e-4d26-bbce-c3520b6c2749\"},{\"content\":{\"connectorIds\":[\"Out1\"],\"side\":\"RIGHT\"},\"type\":\"ConnectorPlacement.EquallySpacedRectSide\",\"uuid\":\"6339fe7c-3981-41e7-9f19-cda16be41a14\"},{\"content\":{\"side\":\"TOP\"},\"type\":\"ConnectorPlacement.EquallySpacedRectSide\",\"uuid\":\"d1729033-563f-49aa-8053-bb4cbe37e0ab\"},{\"content\":{\"connectorIds\":[\"In2\",\"In3\"],\"side\":\"BOTTOM\"},\"type\":\"ConnectorPlacement.EquallySpacedRectSide\",\"uuid\":\"30ea6182-355c-4132-b992-4839827195ad\"}]},\"type\":\"ConnectorPlacement.EquallySpacedConnector\",\"uuid\":\"fc0bd660-6248-4e50-8baf-5497ce638304\"}],\"packageUris\":[\"http://schema.mathworks.com/mf0/Connector/R2020b\"],\"version\":\"1.0\"}"
  Vref1 : InportShadow  Port=3
  VabcRef1 : Outport
  VabcRef : Outport  Port=2
  wires:
  Vabc/1 -> Subsystem1/1
  Vref/1 -> Subsystem1/3
  F/1 -> Subsystem1/2
  Vabc1/1 -> Subsystem2/1
  Vref1/1 -> Subsystem2/3
  F1/1 -> Subsystem2/2
  Subsystem1/1 -> VabcRef/1
  Subsystem2/1 -> VabcRef1/1

== system HVDCMTGW/HVDC STATION  6/Subsystem3 ==
  Vabc1 : Inport
  Vabc : Inport  Port=2
  Vref : Inport  Port=3
  F : Inport  Port=4
  F1 : InportShadow  Port=4
  Subsystem1 : Subsystem  ReferencedSubsystem=WFController  Kpv=offshoregfm.kvp  Kiv=offshoregfm.kvi  Kpicd=offshoregfm.kip  Kiicd=offshoregfm.kii  Kpicq=offshoregfm.kip  Kiicq=offshoregfm.kii  mVAbase=base.mVA  frequency=Grid.frequency  zBase=base.z  iMax=offshoregfm.Imax  L=HVDC.L/5  Kv=base.kV1
      settings: PortSchema="{\"entries\":[{\"content\":{\"sides\":[{\"content\":{\"connectorIds\":[\"In1\"]},\"type\":\"ConnectorPlacement.EquallySpacedRectSide\",\"uuid\":\"46af9a47-930e-4d26-bbce-c3520b6c2749\"},{\"content\":{\"connectorIds\":[\"Out1\"],\"side\":\"RIGHT\"},\"type\":\"ConnectorPlacement.EquallySpacedRectSide\",\"uuid\":\"6339fe7c-3981-41e7-9f19-cda16be41a14\"},{\"content\":{\"side\":\"TOP\"},\"type\":\"ConnectorPlacement.EquallySpacedRectSide\",\"uuid\":\"d1729033-563f-49aa-8053-bb4cbe37e0ab\"},{\"content\":{\"connectorIds\":[\"In2\",\"In3\"],\"side\":\"BOTTOM\"},\"type\":\"ConnectorPlacement.EquallySpacedRectSide\",\"uuid\":\"30ea6182-355c-4132-b992-4839827195ad\"}]},\"type\":\"ConnectorPlacement.EquallySpacedConnector\",\"uuid\":\"fc0bd660-6248-4e50-8baf-5497ce638304\"}],\"packageUris\":[\"http://schema.mathworks.com/mf0/Connector/R2020b\"],\"version\":\"1.0\"}"
  Subsystem2 : Subsystem  ReferencedSubsystem=WFController  Kpv=offshoregfm.kvp  Kiv=offshoregfm.kvi  Kpicd=offshoregfm.kip  Kiicd=offshoregfm.kii  Kpicq=offshoregfm.kip  Kiicq=offshoregfm.kii  mVAbase=base.mVA  frequency=Grid.frequency  zBase=base.z  iMax=offshoregfm.Imax  L=HVDC.L/5  Kv=base.kV1
      settings: PortSchema="{\"entries\":[{\"content\":{\"sides\":[{\"content\":{\"connectorIds\":[\"In1\"]},\"type\":\"ConnectorPlacement.EquallySpacedRectSide\",\"uuid\":\"46af9a47-930e-4d26-bbce-c3520b6c2749\"},{\"content\":{\"connectorIds\":[\"Out1\"],\"side\":\"RIGHT\"},\"type\":\"ConnectorPlacement.EquallySpacedRectSide\",\"uuid\":\"6339fe7c-3981-41e7-9f19-cda16be41a14\"},{\"content\":{\"side\":\"TOP\"},\"type\":\"ConnectorPlacement.EquallySpacedRectSide\",\"uuid\":\"d1729033-563f-49aa-8053-bb4cbe37e0ab\"},{\"content\":{\"connectorIds\":[\"In2\",\"In3\"],\"side\":\"BOTTOM\"},\"type\":\"ConnectorPlacement.EquallySpacedRectSide\",\"uuid\":\"30ea6182-355c-4132-b992-4839827195ad\"}]},\"type\":\"ConnectorPlacement.EquallySpacedConnector\",\"uuid\":\"fc0bd660-6248-4e50-8baf-5497ce638304\"}],\"packageUris\":[\"http://schema.mathworks.com/mf0/Connector/R2020b\"],\"version\":\"1.0\"}"
  Vref1 : InportShadow  Port=3
  VabcRef1 : Outport
  VabcRef : Outport  Port=2
  wires:
  Vabc/1 -> Subsystem1/1
  Vref/1 -> Subsystem1/3
  F/1 -> Subsystem1/2
  Vabc1/1 -> Subsystem2/1
  F1/1 -> Subsystem2/2
  Vref1/1 -> Subsystem2/3
  Subsystem1/1 -> VabcRef/1
  Subsystem2/1 -> VabcRef1/1

== system HVDCMTGW/HVDC STATION 1/Subsystem3 ==
  Current Sensor : fl_lib/Electrical/Electrical Sensors/Current Sensor
  Voltage Sensor1 : fl_lib/Electrical/Electrical Sensors/Voltage Sensor
  - : PMIOPort  Side=Left
  Idc : PMIOPort  Port=2  Side=Right
  Vdc : PMIOPort  Port=3  Side=Right
  + : PMIOPort  Port=4  Side=Right
  Ref : PMIOPort  Port=5  Side=Right
  connections:
  Current Sensor/LConn1 -- +/RConn1 -- Voltage Sensor1/LConn1
  Idc/RConn1 -- Current Sensor/RConn1
  Voltage Sensor1/RConn1 -- Vdc/RConn1
  Voltage Sensor1/RConn2 -- Ref/RConn1
  Current Sensor/RConn2 -- -/RConn1

== system HVDCMTGW/HVDC STATION 2/Subsystem3 ==
  Current Sensor : fl_lib/Electrical/Electrical Sensors/Current Sensor
  Voltage Sensor1 : fl_lib/Electrical/Electrical Sensors/Voltage Sensor
  - : PMIOPort  Side=Left
  Idc : PMIOPort  Port=2  Side=Right
  Vdc : PMIOPort  Port=3  Side=Right
  + : PMIOPort  Port=4  Side=Right
  Ref : PMIOPort  Port=5  Side=Right
  connections:
  Current Sensor/LConn1 -- Voltage Sensor1/LConn1 -- +/RConn1
  Idc/RConn1 -- Current Sensor/RConn1
  Voltage Sensor1/RConn1 -- Vdc/RConn1
  Voltage Sensor1/RConn2 -- Ref/RConn1
  Current Sensor/RConn2 -- -/RConn1

== system HVDCMTGW/HVDC STATION 3/GFL Control ==
  QRef1 : Inport
  QRef : Inport  Port=2
  vdcRef1 : Inport  Port=3
  vdcRef : Inport  Port=4
  PS Terminator : fl_lib/Physical Signals/Sinks/PS Terminator
  Simscape Bus : SimscapeBus  HierarchyStrings=Connection1;Connection2;Connection3
  Simulink-PS Converter1 : nesl_utility/Simulink-PS Converter  PhysicalDomain=network_engine_domain  SubClassName=ps_input  LeftPortType=input  RightPortType=output  PseudoPeriodic=off  Frequencies=[]  NoiseDistribution=none  NoiseParameters=[]  Unit=1  AffineConversion=off  FilteringAndDerivatives=provide  SimscapeFilterOrder=1  InputFilterTimeConstant=0.001  UdotUserProvided=0
  Simulink-PS Converter2 : nesl_utility/Simulink-PS Converter  PhysicalDomain=network_engine_domain  SubClassName=ps_input  LeftPortType=input  RightPortType=output  PseudoPeriodic=off  Frequencies=[]  NoiseDistribution=none  NoiseParameters=[]  Unit=1  AffineConversion=off  FilteringAndDerivatives=provide  SimscapeFilterOrder=1  InputFilterTimeConstant=0.001  UdotUserProvided=0
  Subsystem : Subsystem  ReferencedSubsystem=DCVoltageControl  Kppll=PLL.Kp_pll  Kipll=PLL.Ki_pll  frequency=Grid.frequency  initialPhase=0  sampleTime=-1  Kpicd=PVController.Kp_ic*1.02  Kiicd=PVController.Ki_ic*2  Kdicd=.5  Kpicq=PVController.Kp_ic  Kiicq=PVController.Ki_ic*2  Kdicq=.5  Kpv=20  Kiv=1000  Kdv=0  L=HVDC.L*5  iMax=HVDC.Imaxpu  zBase=Base.z_base  mVAbase=Base.MVA_base_new  VdcBase=HVDC.Vdcbase
  Subsystem1 : Subsystem  ReferencedSubsystem=DCVoltageControl  Kppll=PLL.Kp_pll  Kipll=PLL.Ki_pll  frequency=Grid.frequency  initialPhase=0  sampleTime=-1  Kpicd=PVController.Kp_ic*1.02  Kiicd=PVController.Ki_ic*2  Kdicd=0.5  Kpicq=PVController.Kp_ic  Kiicq=PVController.Ki_ic*2  Kdicq=0.5  Kpv=20  Kiv=1000  Kdv=0  L=HVDC.L*5  iMax=HVDC.Imaxpu  zBase=Base.z_base  mVAbase=Base.MVA_base_new  VdcBase=HVDC.Vdcbase
  Subsystem2 : Subsystem  ReferencedSubsystem=HVDCSTATION  c=HVDC.C*0.175  vc=HVDC.Vdc  L=HVDC.L*100  VRated=Base.KV_base_new  SRated=Base.MVA_base_new  t=Grid.sensor_time  Ts=Ts
  Subsystem3 : Subsystem
  Unit Delay1 : UnitDelay  SampleTime=Ts  HasFrameUpgradeWarning=on
  Unit Delay2 : UnitDelay  SampleTime=Ts  HasFrameUpgradeWarning=on
  DC : PMIOPort  Side=Left
  inv1 : PMIOPort  Port=2  Side=Right
  Idc : PMIOPort  Port=3  Side=Left
  wires:
  Unit Delay1/1 -> Simulink-PS Converter1/1
  Unit Delay2/1 -> Simulink-PS Converter2/1
  Subsystem/1 -> Unit Delay2/1
  Subsystem1/1 -> Unit Delay1/1
  vdcRef/1 -> Subsystem/4
  QRef/1 -> Subsystem/5
  vdcRef1/1 -> Subsystem1/4
  QRef1/1 -> Subsystem1/5
  Subsystem2/1 -> Subsystem/1
  Subsystem2/2 -> Subsystem/2
  Subsystem2/3 -> Subsystem/3
  Subsystem2/4 -> Subsystem1/1
  Subsystem2/5 -> Subsystem1/2
  Subsystem2/6 -> Subsystem1/3
  connections:
  Subsystem2/RConn1 -- inv1/RConn1
  Subsystem2/LConn2 -- Simulink-PS Converter1/RConn1
  Subsystem2/LConn1 -- Simulink-PS Converter2/RConn1
  DC/RConn1 -- Simscape Bus/RConn1
  Simscape Bus/LConn2 -- Subsystem3/RConn4 -- Subsystem2/LConn4
  Idc/RConn1 -- Subsystem3/RConn1
  Subsystem3/RConn3 -- Simscape Bus/LConn1
  Subsystem3/LConn1 -- Subsystem2/LConn3
  PS Terminator/LConn1 -- Subsystem3/RConn2
  Simscape Bus/LConn3 -- Subsystem2/LConn5

== system HVDCMTGW/HVDC STATION 3/GFM Control ==
  QRef1 : Inport
  QRef : Inport  Port=2
  vdcRef1 : Inport  Port=3
  vdcRef : Inport  Port=4
  PS Terminator : fl_lib/Physical Signals/Sinks/PS Terminator
  Simscape Bus : SimscapeBus  HierarchyStrings=Connection1;Connection2;Connection3
  Simulink-PS Converter : nesl_utility/Simulink-PS Converter  PhysicalDomain=network_engine_domain  SubClassName=ps_input  LeftPortType=input  RightPortType=output  PseudoPeriodic=off  Frequencies=[]  NoiseDistribution=none  NoiseParameters=[]  Unit=1  AffineConversion=off  FilteringAndDerivatives=provide  SimscapeFilterOrder=1  InputFilterTimeConstant=0.001  UdotUserProvided=0
  Simulink-PS Converter1 : nesl_utility/Simulink-PS Converter  PhysicalDomain=network_engine_domain  SubClassName=ps_input  LeftPortType=input  RightPortType=output  PseudoPeriodic=off  Frequencies=[]  NoiseDistribution=none  NoiseParameters=[]  Unit=1  AffineConversion=off  FilteringAndDerivatives=provide  SimscapeFilterOrder=1  InputFilterTimeConstant=0.001  UdotUserProvided=0
  Subsystem Reference1 : Subsystem  ReferencedSubsystem=GFMHVDCControllerOnshore  D=onshoreGfm.damping  J=onshoreGfm.inertiaconstant  frequency1=grid.frequency  Pref=onshoreGfm.Pref  kc=onshoreGfm.Evfdroop  Kq=onshoreGfm.QvVdroop  VdRef=onshoreGfm.Vref  Imax1=onshoreGfm.Imax  l=10*HVDC.L/base.z  Kpv=onshoreGfm.Kvp  Kiv=onshoreGfm.Kvi  Vdc=HVDC.Vdc  Kpi=onshoreGfm.Kip  Kii=onshoreGfm.Kii
  Subsystem Reference2 : Subsystem  ReferencedSubsystem=GFMHVDCControllerOnshore  D=onshoreGfm.damping  J=onshoreGfm.inertiaconstant  frequency1=grid.frequency  Pref=onshoreGfm.Pref  kc=onshoreGfm.Evfdroop  Kq=onshoreGfm.QvVdroop  VdRef=onshoreGfm.Vref  Imax1=onshoreGfm.Imax  l=10*HVDC.L/base.z  Kpv=onshoreGfm.Kvp  Kiv=onshoreGfm.Kvi  Vdc=HVDC.Vdc  Kpi=onshoreGfm.Kip  Kii=onshoreGfm.Kii
  Subsystem2 : Subsystem  ReferencedSubsystem=HVDCSTATION  c=HVDC.C  vc=HVDC.Vdc  L=HVDC.L*10  VRated=Base.KV_base_new  SRated=Base.MVA_base_new  t=Grid.sensor_time  Ts=Ts
  Subsystem3 : Subsystem
  Unit Delay : UnitDelay  SampleTime=-1  HasFrameUpgradeWarning=on
  Unit Delay1 : UnitDelay  SampleTime=-1  HasFrameUpgradeWarning=on
  DC : PMIOPort  Side=Left
  inv1 : PMIOPort  Port=2  Side=Right
  Idc : PMIOPort  Port=3  Side=Left
  wires:
  QRef/1 -> Subsystem Reference2/5
  vdcRef/1 -> Subsystem Reference2/4
  vdcRef1/1 -> Subsystem Reference1/4
  QRef1/1 -> Subsystem Reference1/5
  Subsystem2/1 -> Subsystem Reference2/1
  Subsystem2/4 -> Subsystem Reference1/1
  Subsystem2/2 -> Subsystem Reference2/2
  Subsystem2/3 -> Subsystem Reference2/3
  Subsystem2/5 -> Subsystem Reference1/2
  Subsystem2/6 -> Subsystem Reference1/3
  Subsystem Reference2/1 -> Unit Delay/1
  Unit Delay/1 -> Simulink-PS Converter/1
  Subsystem Reference1/1 -> Unit Delay1/1
  Unit Delay1/1 -> Simulink-PS Converter1/1
  connections:
  DC/RConn1 -- Simscape Bus/RConn1
  Idc/RConn1 -- Subsystem3/RConn1
  Subsystem3/RConn3 -- Simscape Bus/LConn1
  Subsystem3/LConn1 -- Subsystem2/LConn3
  Subsystem3/RConn4 -- Subsystem2/LConn4 -- Simscape Bus/LConn2
  Subsystem2/LConn5 -- Simscape Bus/LConn3
  PS Terminator/LConn1 -- Subsystem3/RConn2
  Subsystem2/RConn1 -- inv1/RConn1
  Simulink-PS Converter/RConn1 -- Subsystem2/LConn1
  Simulink-PS Converter1/RConn1 -- Subsystem2/LConn2

== system HVDCMTGW/Wind Farm 1/PLL & Measurements ==
  V : Inport
  Ig : Inport  Port=2
  Measurement1 : Subsystem
  Measurement2 : Subsystem
  PLL : Subsystem
  Out Bus Element : Outport  PortName=Vbus  Element=Vq
  Out Bus Element1 : Outport  PortName=Vbus  Element=Vd
  Out Bus Element2 : Outport  PortName=Vbus  Element=w
  Out Bus Element3 : Outport  PortName=Vbus  Element=Theta
  Out Bus Element4 : Outport  PortName=Vbus  Element=Vmag
  Out Bus Element5 : Outport  PortName=Vbus  Element=Id
  Out Bus Element6 : Outport  PortName=Vbus  Element=Iq
  wires:
  V/1 -> Measurement2/1(u)
  PLL/2(freq) -> Out Bus Element2/1  "w"
  PLL/5(Vq) -> Out Bus Element/1  "Vq"
  PLL/3(angle) -> Out Bus Element3/1
  PLL/4(Vd) -> Out Bus Element1/1  "Vd"
  Measurement2/1(Vg) -> PLL/1(abc)
  PLL/1(mag) -> Out Bus Element4/1  "Vmag"
  Measurement1/1(Ig) -> PLL/2(Ig)
  Ig/1 -> Measurement1/1(u)
  PLL/7(Iq) -> Out Bus Element6/1  "Iq"
  PLL/6(Id) -> Out Bus Element5/1  "Id"

== system HVDCMTGW/Wind Farm 1/Wind Farm ==
  Vbus : Inport
  Abstract : Subsystem  VariantControl=Choice1==2
  Detail : Subsystem  VariantControl=Choice1==1
  abc : PMIOPort  Side=Right
  abc1 : PMIOPort  Port=2  Side=Right
  Vabc : Outport
  Iabc : Outport  Port=2

== system HVDCMTGW/Wind Farm 2/PLL & Measurements ==
  V : Inport
  Ig : Inport  Port=2
  Measurement1 : Subsystem
  Measurement2 : Subsystem
  PLL : Subsystem
  Out Bus Element : Outport  PortName=Vbus  Element=Vq
  Out Bus Element1 : Outport  PortName=Vbus  Element=Vd
  Out Bus Element2 : Outport  PortName=Vbus  Element=w
  Out Bus Element3 : Outport  PortName=Vbus  Element=Theta
  Out Bus Element4 : Outport  PortName=Vbus  Element=Vmag
  Out Bus Element5 : Outport  PortName=Vbus  Element=Id
  Out Bus Element6 : Outport  PortName=Vbus  Element=Iq
  wires:
  V/1 -> Measurement2/1(u)
  PLL/2(freq) -> Out Bus Element2/1  "w"
  PLL/5(Vq) -> Out Bus Element/1  "Vq"
  PLL/3(angle) -> Out Bus Element3/1
  PLL/4(Vd) -> Out Bus Element1/1  "Vd"
  Measurement2/1(Vg) -> PLL/1(abc)
  PLL/1(mag) -> Out Bus Element4/1  "Vmag"
  Measurement1/1(Ig) -> PLL/2(Ig)
  Ig/1 -> Measurement1/1(u)
  PLL/7(Iq) -> Out Bus Element6/1  "Iq"
  PLL/6(Id) -> Out Bus Element5/1  "Id"

== system HVDCMTGW/Wind Farm 2/Wind Farm ==
  Vbus : Inport
  Abstract : Subsystem  VariantControl=Choice1==2
  Detail : Subsystem  VariantControl=Choice1==1
  abc : PMIOPort  Side=Right
  abc1 : PMIOPort  Port=2  Side=Right
  Vabc : Outport
  Iabc : Outport  Port=2

== system HVDCMTGW/HVDC STATION 3/GFL Control/Subsystem3 ==
  Current Sensor : fl_lib/Electrical/Electrical Sensors/Current Sensor
  Voltage Sensor1 : fl_lib/Electrical/Electrical Sensors/Voltage Sensor
  - : PMIOPort  Side=Left
  Idc : PMIOPort  Port=2  Side=Right
  Vdc : PMIOPort  Port=3  Side=Right
  + : PMIOPort  Port=4  Side=Right
  Ref : PMIOPort  Port=5  Side=Right
  connections:
  Current Sensor/LConn1 -- Voltage Sensor1/LConn1 -- +/RConn1
  Idc/RConn1 -- Current Sensor/RConn1
  Voltage Sensor1/RConn1 -- Vdc/RConn1
  Voltage Sensor1/RConn2 -- Ref/RConn1
  Current Sensor/RConn2 -- -/RConn1
